simulink model "dualArrayTask"  (R2012b)
settings: Solver=FixedStepDiscrete  SolverMode=MultiTasking  StartTime=0.0  StopTime=10.0  FixedStep=0.001  RelTol=1e-3
settings Model: xpc_rtwmakecfg_data=_xpcetherlib__xpcether8255xlib__xpcetherGbElib__xpcnblib_  BufferReuse=off  Creator=gilja  LastModifiedBy=NPTL
settings SolverCC: EnableConcurrentExecution=on  ConcurrentTasks=on
settings DataIOCC: SaveOutput=off  SignalLogging=off  DSMLogging=off  SaveTime=off
settings OptimizationCC: BlockReduction=off  InlineParams=on  InlineInvariantSignals=on  OptimizeBlockIOStorage=off  BufferReuse=off  ExpressionFolding=off  LocalBlockOutputs=off
settings HardwareCC: ProdIntDivRoundTo=Zero  ProdEndianess=LittleEndian  ProdHWDeviceType=Generic->32-bit x86 compatible
settings ModelReferenceCC: ModelReferenceNumInstancesAllowed=Single  PropagateVarSize=During execution  ModelReferenceMinAlgLoopOccurrences=on
settings RTWCC: SystemTargetFile=xpctarget.tlc  TemplateMakefile=xpc_default_tmf  Description=xPC Target  ProcessScript=xpctarget_make_rtw_hook  RTWCompilerOptimization=On
settings CodeAppCC: MaxIdLength=62
settings xpcTargetCC: TargetFcnLib=ansi_tfl_table_tmw.mat  CodeReplacementLibrary=XPC_BLAS  ParMdlRefBuildCompliant=on  ConcurrentExecutionCompliant=on  CombineSignalStateStructs=off  GRTInterface=on  xPCTaskExecutionProfile=on  xPCRL32EventNumber=5000  xPCisDownloadable=off  xPCLoadParamSetFile=off  xPCConcurrentTasks=off  xPCEnableSFAnimation=off

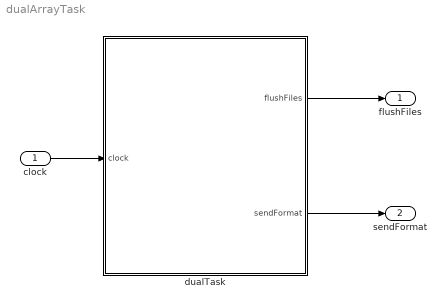
== system dualArrayTask ==
  clock : Inport  OutDataTypeStr=uint32
  dualTask : MATLAB Function  TreatAsAtomicUnit=on
  flushFiles : Outport  BusOutputAsStruct=on
  sendFormat : Outport  Port=2  BusOutputAsStruct=on
  wires:
  dualTask/1(flushFiles) -> flushFiles/1
  clock/1 -> dualTask/1(clock)
  dualTask/2(sendFormat) -> sendFormat/1

== matlab function dualArrayTask/dualTask ==
  data: flushFiles output size=1; clock input; sendFormat output
function [flushFiles, sendFormat] = dualTask(clock)

flushFiles = false;
sendFormat = false;

% if clock == 200
%     flushFiles = true;
% end
% 
if clock>200 && clock < 1000 && mod(clock,100)==0
    sendFormat = true;
end
